simulink model "Unknown_Terrain_BOTS"  (R2018b)
settings: Solver=VariableStepAuto  StartTime=0.0  StopTime=10.0  RelTol=1e-3
model workspace: external: MATLAB File F:\Projects\Relative Localiztion\CAD models\Simulation\Unknown_Terrain_BOTS_DataFile.m (data not in the file)
values from neighbouring files (symbols this model uses):
  BOT1_pos = zeros(3,length(t))    [Tetrahedron_Based_Relative_Localization.m]
  bot1_transmitted = zeros(3,length(t))    [Transmission_Channal.m]
  BOT2_pos = zeros(3,length(t))    [Tetrahedron_Based_Relative_Localization.m]
  bot2_transmitted = zeros(3,length(t))    [Transmission_Channal.m]
  BOT3_pos = zeros(3,length(t))    [Tetrahedron_Based_Relative_Localization.m]
  bot3_transmitted = zeros(3,length(t))    [Transmission_Channal.m]
  BOT4_pos = zeros(3,length(t))    [Tetrahedron_Based_Relative_Localization.m]
  bot4_transmitted = zeros(3,length(t))    [Transmission_Channal.m]
undefined symbols (not defined in the file or in its folder): smiData, X, Y, Z
libraries: simulink x60, sm_lib x29, nesl_utility x25
(part 2 of 2)

== system Unknown_Terrain_BOTS/BOT1/BOT1_RIGID ==
  ReferenceFrame : sm_lib/Frames and Transforms/Reference Frame
  Solid : sm_lib/Body Elements/Solid  InertiaType=Custom  Mass=smiData.Solid(3).mass  MassUnits=kg  CenterOfMass=smiData.Solid(3).CoM  CenterOfMassUnits=mm  MomentsOfInertia=smiData.Solid(3).MoI  MomentsOfInertiaUnits=kg*mm^2  ProductsOfInertia=smiData.Solid(3).PoI  ProductsOfInertiaUnits=kg*mm^2  BasedOnType=Density  Density=1000  DensityUnits=kg/m^3  DoExposeReferenceFrame=on  SerializedFrames=<Frames/>  GraphicType=FromGeometry  MarkerShape=Sphere  MarkerSize=10  GraphicVisPropType=AdvancedVisualProperties  GraphicDiffuseColor=[1.0 0.2 0.2]  GraphicSpecularColor=[0.5 0.5 0.5 1.0]  GraphicAmbientColor=[0.15 0.15 0.15 1.0]  GraphicEmissiveColor=[0.0 0.0 0.0 1.0]  GraphicShininess=75  GraphicOpacity=smiData.Solid(3).opacity  GeometryShape=FromFile  RectangleSize=[1 1]  RectangleSizeUnits=m  BrickDimensions=[1 1 1]  BrickDimensionUnits=m  CylinderRadius=1  CylinderRadiusUnits=m  CylinderLength=1  CylinderLengthUnits=m  SphereRadius=1  SphereRadiusUnits=m  EllipsoidRadii=[1 1 1]  EllipsoidRadiiUnits=m  ExtrusionCrossSection=[1 1; -1 1; -1 -1; 1 -1]  ExtrusionCrossSectionUnits=m  ExtrusionLength=1  ExtrusionLengthUnits=m  PolygonNumSides=3  PolygonOuterRadius=1  PolygonOuterRadiusUnits=m  ExtGeomFileType=STEP  ExtGeomFileName=BOT3_Default_sldprt.STEP  ExtGeomFileUnits=m  RevolutionCrossSection=[1 1; 1 -1; 2 -1; 2 1]  RevolutionCrossSectionUnits=m  RevolutionExtent=Full  RevolutionAngle=180  RevolutionAngleUnits=deg
  Transform : sm_lib/Frames and Transforms/Rigid Transform  TranslationMethod=Cartesian  TranslationStandardOffset=0  TranslationLengthUnit=m  TranslationStandardAxis=+Z  TranslationCartesianOffset=smiData.RigidTransform(6).translation  TranslationROffset=0  TranslationROffsetUnits=m  TranslationZOffset=0  TranslationZOffsetUnits=m  TranslationThetaOffset=0  TranslationThetaOffsetUnits=deg  RotationMethod=ArbitraryAxis  RotationAngleUnits=rad  RotationStandardAxis=+Z  RotationAngle=smiData.RigidTransform(6).angle  RotationArbitraryAxis=smiData.RigidTransform(6).axis  FollAlignAxisA=+X  BaseAlignAxisA=+Y  FollAlignAxisB=+Y  BaseAlignAxisB=+Z  RotationSequenceAxes=FollowerAxes  RotationSequence=XYX  RotationSequenceAngles=[0 0 0]  RotationSequenceAnglesUnits=deg  RotationMatrix=[1 0 0; 0 1 0; 0 0 1]
  F : PMIOPort  Side=Left
  connections:
  Solid/RConn1 -- ReferenceFrame/RConn1 -- Transform/LConn1
  Transform/RConn1 -- F/RConn1

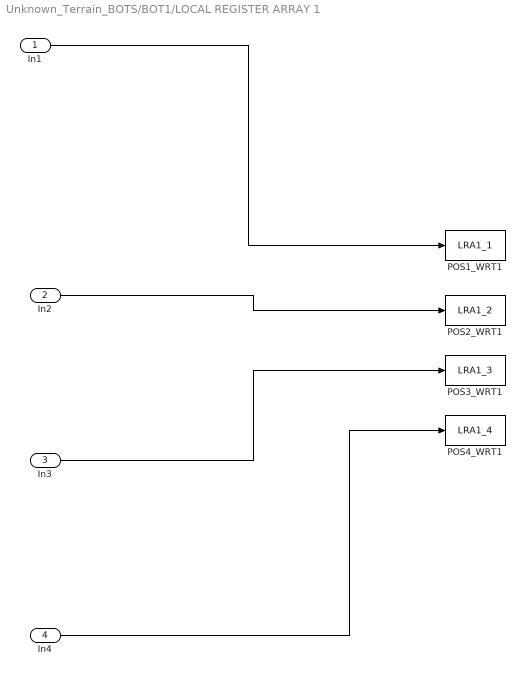
== system Unknown_Terrain_BOTS/BOT1/LOCAL REGISTER ARRAY 1 ==
  In1 : Inport
  In2 : Inport  Port=2
  In3 : Inport  Port=3
  In4 : Inport  Port=4
  POS1_WRT1 : ToWorkspace  VariableName=LRA1_1  SampleTime=-1
  POS2_WRT1 : ToWorkspace  VariableName=LRA1_2  SampleTime=-1
  POS3_WRT1 : ToWorkspace  VariableName=LRA1_3  SampleTime=-1
  POS4_WRT1 : ToWorkspace  VariableName=LRA1_4  SampleTime=-1
  wires:
  In2/1 -> POS2_WRT1/1
  In3/1 -> POS3_WRT1/1
  In1/1 -> POS1_WRT1/1
  In4/1 -> POS4_WRT1/1

== system Unknown_Terrain_BOTS/BOT1/Subsystem ==
  1 : Inport
  Gain : Gain  Gain=-1
  Sum : Sum  Inputs=|++
  z0 : Constant  Value=0.2889717
  2 : Outport
  wires:
  z0/1 -> Sum/2
  Gain/1 -> Sum/1
  Sum/1 -> 2/1
  1/1 -> Gain/1

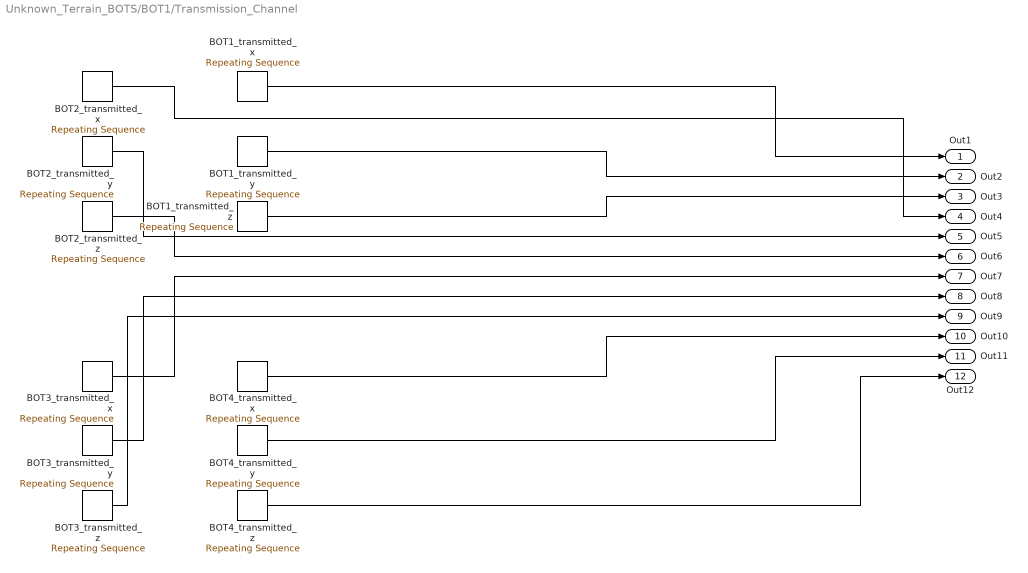
== system Unknown_Terrain_BOTS/BOT1/Transmission_Channel ==
  BOT1_transmitted_x : simulink/Sources/Repeating Sequence  rep_seq_t=t  rep_seq_y=bot1_transmitted(1,:)
  BOT1_transmitted_y : simulink/Sources/Repeating Sequence  rep_seq_t=t  rep_seq_y=bot1_transmitted(2,:)
  BOT1_transmitted_z : simulink/Sources/Repeating Sequence  rep_seq_t=t  rep_seq_y=bot1_transmitted(3,:)
  BOT2_transmitted_x : simulink/Sources/Repeating Sequence  rep_seq_t=t  rep_seq_y=bot2_transmitted(1,:)
  BOT2_transmitted_y : simulink/Sources/Repeating Sequence  rep_seq_t=t  rep_seq_y=bot2_transmitted(2,:)
  BOT2_transmitted_z : simulink/Sources/Repeating Sequence  rep_seq_t=t  rep_seq_y=bot2_transmitted(3,:)
  BOT3_transmitted_x : simulink/Sources/Repeating Sequence  rep_seq_t=t  rep_seq_y=bot3_transmitted(1,:)
  BOT3_transmitted_y : simulink/Sources/Repeating Sequence  rep_seq_t=t  rep_seq_y=bot3_transmitted(2,:)
  BOT3_transmitted_z : simulink/Sources/Repeating Sequence  rep_seq_t=t  rep_seq_y=bot3_transmitted(3,:)
  BOT4_transmitted_x : simulink/Sources/Repeating Sequence  rep_seq_t=t  rep_seq_y=bot4_transmitted(1,:)
  BOT4_transmitted_y : simulink/Sources/Repeating Sequence  rep_seq_t=t  rep_seq_y=bot4_transmitted(2,:)
  BOT4_transmitted_z : simulink/Sources/Repeating Sequence  rep_seq_t=t  rep_seq_y=bot4_transmitted(3,:)
  Out1 : Outport
  Out2 : Outport  Port=2
  Out3 : Outport  Port=3
  Out4 : Outport  Port=4
  Out5 : Outport  Port=5
  Out6 : Outport  Port=6
  Out7 : Outport  Port=7
  Out8 : Outport  Port=8
  Out9 : Outport  Port=9
  Out10 : Outport  Port=10
  Out11 : Outport  Port=11
  Out12 : Outport  Port=12
  wires:
  BOT1_transmitted_x/1 -> Out1/1
  BOT4_transmitted_z/1 -> Out12/1
  BOT1_transmitted_z/1 -> Out3/1
  BOT3_transmitted_x/1 -> Out7/1
  BOT3_transmitted_z/1 -> Out9/1
  BOT2_transmitted_z/1 -> Out6/1
  BOT2_transmitted_y/1 -> Out5/1
  BOT3_transmitted_y/1 -> Out8/1
  BOT1_transmitted_y/1 -> Out2/1
  BOT2_transmitted_x/1 -> Out4/1
  BOT4_transmitted_x/1 -> Out10/1
  BOT4_transmitted_y/1 -> Out11/1

== system Unknown_Terrain_BOTS/BOT2/BOT2_RIGID ==
  ReferenceFrame : sm_lib/Frames and Transforms/Reference Frame
  Solid : sm_lib/Body Elements/Solid  InertiaType=Custom  Mass=smiData.Solid(4).mass  MassUnits=kg  CenterOfMass=smiData.Solid(4).CoM  CenterOfMassUnits=mm  MomentsOfInertia=smiData.Solid(4).MoI  MomentsOfInertiaUnits=kg*mm^2  ProductsOfInertia=smiData.Solid(4).PoI  ProductsOfInertiaUnits=kg*mm^2  BasedOnType=Density  Density=1000  DensityUnits=kg/m^3  DoExposeReferenceFrame=on  SerializedFrames=<Frames/>  GraphicType=FromGeometry  MarkerShape=Sphere  MarkerSize=10  GraphicVisPropType=AdvancedVisualProperties  GraphicDiffuseColor=[0.6 1.0 0.2]  GraphicSpecularColor=[0.5 0.5 0.5 1.0]  GraphicAmbientColor=[0.15 0.15 0.15 1.0]  GraphicEmissiveColor=[0.0 0.0 0.0 1.0]  GraphicShininess=75  GraphicOpacity=smiData.Solid(4).opacity  GeometryShape=FromFile  RectangleSize=[1 1]  RectangleSizeUnits=m  BrickDimensions=[1 1 1]  BrickDimensionUnits=m  CylinderRadius=1  CylinderRadiusUnits=m  CylinderLength=1  CylinderLengthUnits=m  SphereRadius=1  SphereRadiusUnits=m  EllipsoidRadii=[1 1 1]  EllipsoidRadiiUnits=m  ExtrusionCrossSection=[1 1; -1 1; -1 -1; 1 -1]  ExtrusionCrossSectionUnits=m  ExtrusionLength=1  ExtrusionLengthUnits=m  PolygonNumSides=3  PolygonOuterRadius=1  PolygonOuterRadiusUnits=m  ExtGeomFileType=STEP  ExtGeomFileName=BOT4_Default_sldprt.STEP  ExtGeomFileUnits=m  RevolutionCrossSection=[1 1; 1 -1; 2 -1; 2 1]  RevolutionCrossSectionUnits=m  RevolutionExtent=Full  RevolutionAngle=180  RevolutionAngleUnits=deg
  Transform : sm_lib/Frames and Transforms/Rigid Transform  TranslationMethod=Cartesian  TranslationStandardOffset=0  TranslationLengthUnit=m  TranslationStandardAxis=+Z  TranslationCartesianOffset=smiData.RigidTransform(8).translation  TranslationROffset=0  TranslationROffsetUnits=m  TranslationZOffset=0  TranslationZOffsetUnits=m  TranslationThetaOffset=0  TranslationThetaOffsetUnits=deg  RotationMethod=ArbitraryAxis  RotationAngleUnits=rad  RotationStandardAxis=+Z  RotationAngle=smiData.RigidTransform(8).angle  RotationArbitraryAxis=smiData.RigidTransform(8).axis  FollAlignAxisA=+X  BaseAlignAxisA=+Y  FollAlignAxisB=+Y  BaseAlignAxisB=+Z  RotationSequenceAxes=FollowerAxes  RotationSequence=XYX  RotationSequenceAngles=[0 0 0]  RotationSequenceAnglesUnits=deg  RotationMatrix=[1 0 0; 0 1 0; 0 0 1]
  F : PMIOPort  Side=Left
  connections:
  Solid/RConn1 -- ReferenceFrame/RConn1 -- Transform/LConn1
  Transform/RConn1 -- F/RConn1

== system Unknown_Terrain_BOTS/BOT2/LOCAL REGISTER ARRAY 2 ==
  In1 : Inport
  In2 : Inport  Port=2
  In3 : Inport  Port=3
  In4 : Inport  Port=4
  POS1_WRT2 : ToWorkspace  VariableName=LRA2_1  SampleTime=-1
  POS2_WRT2 : ToWorkspace  VariableName=LRA2_2  SampleTime=-1
  POS3_WRT2 : ToWorkspace  VariableName=LRA2_3  SampleTime=-1
  POS4_WRT2 : ToWorkspace  VariableName=LRA2_4  SampleTime=-1
  wires:
  In2/1 -> POS2_WRT2/1
  In3/1 -> POS3_WRT2/1
  In1/1 -> POS1_WRT2/1
  In4/1 -> POS4_WRT2/1

== system Unknown_Terrain_BOTS/BOT2/Subsystem ==
  1 : Inport
  Gain : Gain
  Sum : Sum  Inputs=|++
  z0 : Constant  Value=-0.2889717
  2 : Outport
  wires:
  z0/1 -> Sum/2
  Gain/1 -> Sum/1
  Sum/1 -> 2/1
  1/1 -> Gain/1

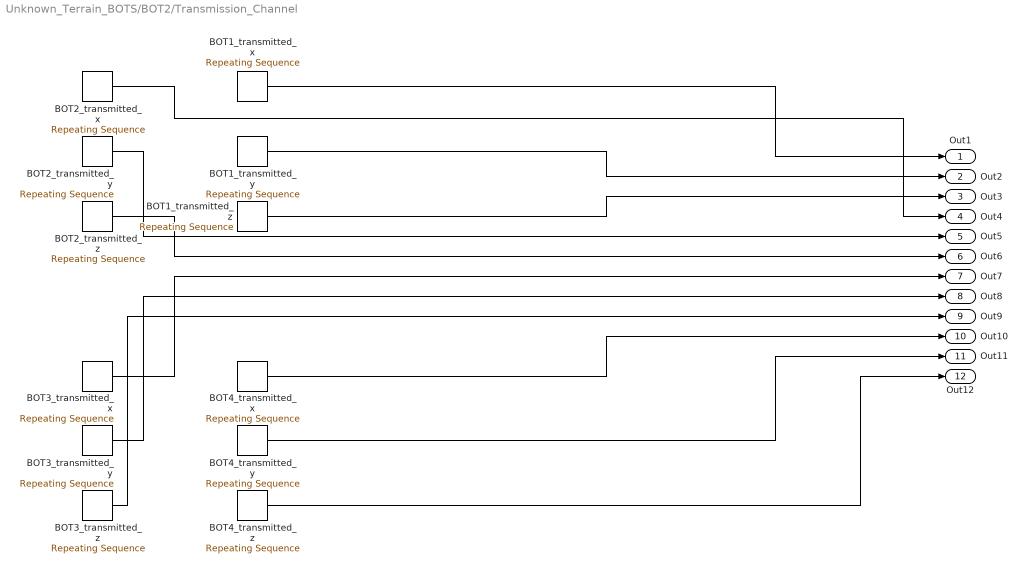
== system Unknown_Terrain_BOTS/BOT2/Transmission_Channel ==
  BOT1_transmitted_x : simulink/Sources/Repeating Sequence  rep_seq_t=t  rep_seq_y=bot1_transmitted(1,:)
  BOT1_transmitted_y : simulink/Sources/Repeating Sequence  rep_seq_t=t  rep_seq_y=bot1_transmitted(2,:)
  BOT1_transmitted_z : simulink/Sources/Repeating Sequence  rep_seq_t=t  rep_seq_y=bot1_transmitted(3,:)
  BOT2_transmitted_x : simulink/Sources/Repeating Sequence  rep_seq_t=t  rep_seq_y=bot2_transmitted(1,:)
  BOT2_transmitted_y : simulink/Sources/Repeating Sequence  rep_seq_t=t  rep_seq_y=bot2_transmitted(2,:)
  BOT2_transmitted_z : simulink/Sources/Repeating Sequence  rep_seq_t=t  rep_seq_y=bot2_transmitted(3,:)
  BOT3_transmitted_x : simulink/Sources/Repeating Sequence  rep_seq_t=t  rep_seq_y=bot3_transmitted(1,:)
  BOT3_transmitted_y : simulink/Sources/Repeating Sequence  rep_seq_t=t  rep_seq_y=bot3_transmitted(2,:)
  BOT3_transmitted_z : simulink/Sources/Repeating Sequence  rep_seq_t=t  rep_seq_y=bot3_transmitted(3,:)
  BOT4_transmitted_x : simulink/Sources/Repeating Sequence  rep_seq_t=t  rep_seq_y=bot4_transmitted(1,:)
  BOT4_transmitted_y : simulink/Sources/Repeating Sequence  rep_seq_t=t  rep_seq_y=bot4_transmitted(2,:)
  BOT4_transmitted_z : simulink/Sources/Repeating Sequence  rep_seq_t=t  rep_seq_y=bot4_transmitted(3,:)
  Out1 : Outport
  Out2 : Outport  Port=2
  Out3 : Outport  Port=3
  Out4 : Outport  Port=4
  Out5 : Outport  Port=5
  Out6 : Outport  Port=6
  Out7 : Outport  Port=7
  Out8 : Outport  Port=8
  Out9 : Outport  Port=9
  Out10 : Outport  Port=10
  Out11 : Outport  Port=11
  Out12 : Outport  Port=12
  wires:
  BOT1_transmitted_x/1 -> Out1/1
  BOT4_transmitted_z/1 -> Out12/1
  BOT1_transmitted_z/1 -> Out3/1
  BOT3_transmitted_x/1 -> Out7/1
  BOT3_transmitted_z/1 -> Out9/1
  BOT2_transmitted_z/1 -> Out6/1
  BOT2_transmitted_y/1 -> Out5/1
  BOT3_transmitted_y/1 -> Out8/1
  BOT1_transmitted_y/1 -> Out2/1
  BOT2_transmitted_x/1 -> Out4/1
  BOT4_transmitted_x/1 -> Out10/1
  BOT4_transmitted_y/1 -> Out11/1

== system Unknown_Terrain_BOTS/BOT3/BOT3_RIGID ==
  ReferenceFrame : sm_lib/Frames and Transforms/Reference Frame
  Solid : sm_lib/Body Elements/Solid  InertiaType=Custom  Mass=smiData.Solid(2).mass  MassUnits=kg  CenterOfMass=smiData.Solid(2).CoM  CenterOfMassUnits=mm  MomentsOfInertia=smiData.Solid(2).MoI  MomentsOfInertiaUnits=kg*mm^2  ProductsOfInertia=smiData.Solid(2).PoI  ProductsOfInertiaUnits=kg*mm^2  BasedOnType=Density  Density=1000  DensityUnits=kg/m^3  DoExposeReferenceFrame=on  SerializedFrames=<Frames/>  GraphicType=FromGeometry  MarkerShape=Sphere  MarkerSize=10  GraphicVisPropType=AdvancedVisualProperties  GraphicDiffuseColor=[0.0 0.2 1.0]  GraphicSpecularColor=[0.5 0.5 0.5 1.0]  GraphicAmbientColor=[0.15 0.15 0.15 1.0]  GraphicEmissiveColor=[0.0 0.0 0.0 1.0]  GraphicShininess=75  GraphicOpacity=smiData.Solid(2).opacity  GeometryShape=FromFile  RectangleSize=[1 1]  RectangleSizeUnits=m  BrickDimensions=[1 1 1]  BrickDimensionUnits=m  CylinderRadius=1  CylinderRadiusUnits=m  CylinderLength=1  CylinderLengthUnits=m  SphereRadius=1  SphereRadiusUnits=m  EllipsoidRadii=[1 1 1]  EllipsoidRadiiUnits=m  ExtrusionCrossSection=[1 1; -1 1; -1 -1; 1 -1]  ExtrusionCrossSectionUnits=m  ExtrusionLength=1  ExtrusionLengthUnits=m  PolygonNumSides=3  PolygonOuterRadius=1  PolygonOuterRadiusUnits=m  ExtGeomFileType=STEP  ExtGeomFileName=BOT2_Default_sldprt.STEP  ExtGeomFileUnits=m  RevolutionCrossSection=[1 1; 1 -1; 2 -1; 2 1]  RevolutionCrossSectionUnits=m  RevolutionExtent=Full  RevolutionAngle=180  RevolutionAngleUnits=deg
  Transform : sm_lib/Frames and Transforms/Rigid Transform  TranslationMethod=Cartesian  TranslationStandardOffset=0  TranslationLengthUnit=m  TranslationStandardAxis=+Z  TranslationCartesianOffset=smiData.RigidTransform(4).translation  TranslationROffset=0  TranslationROffsetUnits=m  TranslationZOffset=0  TranslationZOffsetUnits=m  TranslationThetaOffset=0  TranslationThetaOffsetUnits=deg  RotationMethod=ArbitraryAxis  RotationAngleUnits=rad  RotationStandardAxis=+Z  RotationAngle=smiData.RigidTransform(4).angle  RotationArbitraryAxis=smiData.RigidTransform(4).axis  FollAlignAxisA=+X  BaseAlignAxisA=+Y  FollAlignAxisB=+Y  BaseAlignAxisB=+Z  RotationSequenceAxes=FollowerAxes  RotationSequence=XYX  RotationSequenceAngles=[0 0 0]  RotationSequenceAnglesUnits=deg  RotationMatrix=[1 0 0; 0 1 0; 0 0 1]
  F : PMIOPort  Side=Left
  connections:
  Solid/RConn1 -- ReferenceFrame/RConn1 -- Transform/LConn1
  Transform/RConn1 -- F/RConn1

== system Unknown_Terrain_BOTS/BOT3/LOCAL REGISTER ARRAY 3 ==
  In1 : Inport
  In2 : Inport  Port=2
  In3 : Inport  Port=3
  In4 : Inport  Port=4
  POS1_WRT3 : ToWorkspace  VariableName=LRA3_1  SampleTime=-1
  POS2_WRT3 : ToWorkspace  VariableName=LRA3_2  SampleTime=-1
  POS3_WRT3 : ToWorkspace  VariableName=LRA3_3  SampleTime=-1
  POS4_WRT3 : ToWorkspace  VariableName=LRA3_4  SampleTime=-1
  wires:
  In2/1 -> POS2_WRT3/1
  In3/1 -> POS3_WRT3/1
  In1/1 -> POS1_WRT3/1
  In4/1 -> POS4_WRT3/1

== system Unknown_Terrain_BOTS/BOT3/Subsystem ==
  1 : Inport
  Gain : Gain
  Sum : Sum  Inputs=|++
  z0 : Constant  Value=-0.2889717
  2 : Outport
  wires:
  z0/1 -> Sum/2
  Gain/1 -> Sum/1
  Sum/1 -> 2/1
  1/1 -> Gain/1

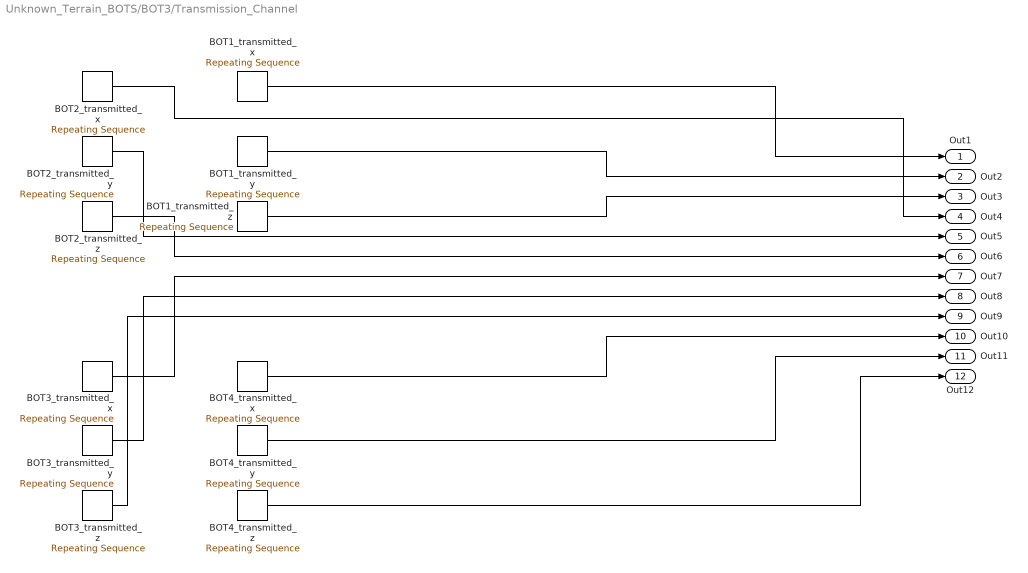
== system Unknown_Terrain_BOTS/BOT3/Transmission_Channel ==
  BOT1_transmitted_x : simulink/Sources/Repeating Sequence  rep_seq_t=t  rep_seq_y=bot1_transmitted(1,:)
  BOT1_transmitted_y : simulink/Sources/Repeating Sequence  rep_seq_t=t  rep_seq_y=bot1_transmitted(2,:)
  BOT1_transmitted_z : simulink/Sources/Repeating Sequence  rep_seq_t=t  rep_seq_y=bot1_transmitted(3,:)
  BOT2_transmitted_x : simulink/Sources/Repeating Sequence  rep_seq_t=t  rep_seq_y=bot2_transmitted(1,:)
  BOT2_transmitted_y : simulink/Sources/Repeating Sequence  rep_seq_t=t  rep_seq_y=bot2_transmitted(2,:)
  BOT2_transmitted_z : simulink/Sources/Repeating Sequence  rep_seq_t=t  rep_seq_y=bot2_transmitted(3,:)
  BOT3_transmitted_x : simulink/Sources/Repeating Sequence  rep_seq_t=t  rep_seq_y=bot3_transmitted(1,:)
  BOT3_transmitted_y : simulink/Sources/Repeating Sequence  rep_seq_t=t  rep_seq_y=bot3_transmitted(2,:)
  BOT3_transmitted_z : simulink/Sources/Repeating Sequence  rep_seq_t=t  rep_seq_y=bot3_transmitted(3,:)
  BOT4_transmitted_x : simulink/Sources/Repeating Sequence  rep_seq_t=t  rep_seq_y=bot4_transmitted(1,:)
  BOT4_transmitted_y : simulink/Sources/Repeating Sequence  rep_seq_t=t  rep_seq_y=bot4_transmitted(2,:)
  BOT4_transmitted_z : simulink/Sources/Repeating Sequence  rep_seq_t=t  rep_seq_y=bot4_transmitted(3,:)
  Out1 : Outport
  Out2 : Outport  Port=2
  Out3 : Outport  Port=3
  Out4 : Outport  Port=4
  Out5 : Outport  Port=5
  Out6 : Outport  Port=6
  Out7 : Outport  Port=7
  Out8 : Outport  Port=8
  Out9 : Outport  Port=9
  Out10 : Outport  Port=10
  Out11 : Outport  Port=11
  Out12 : Outport  Port=12
  wires:
  BOT1_transmitted_x/1 -> Out1/1
  BOT4_transmitted_z/1 -> Out12/1
  BOT1_transmitted_z/1 -> Out3/1
  BOT3_transmitted_x/1 -> Out7/1
  BOT3_transmitted_z/1 -> Out9/1
  BOT2_transmitted_z/1 -> Out6/1
  BOT2_transmitted_y/1 -> Out5/1
  BOT3_transmitted_y/1 -> Out8/1
  BOT1_transmitted_y/1 -> Out2/1
  BOT2_transmitted_x/1 -> Out4/1
  BOT4_transmitted_x/1 -> Out10/1
  BOT4_transmitted_y/1 -> Out11/1

== system Unknown_Terrain_BOTS/BOT4/BOT4_RIGID ==
  ReferenceFrame : sm_lib/Frames and Transforms/Reference Frame
  Solid : sm_lib/Body Elements/Solid  InertiaType=Custom  Mass=smiData.Solid(1).mass  MassUnits=kg  CenterOfMass=smiData.Solid(1).CoM  CenterOfMassUnits=mm  MomentsOfInertia=smiData.Solid(1).MoI  MomentsOfInertiaUnits=kg*mm^2  ProductsOfInertia=smiData.Solid(1).PoI  ProductsOfInertiaUnits=kg*mm^2  BasedOnType=Density  Density=1000  DensityUnits=kg/m^3  DoExposeReferenceFrame=on  SerializedFrames=<Frames/>  GraphicType=FromGeometry  MarkerShape=Sphere  MarkerSize=10  GraphicVisPropType=AdvancedVisualProperties  GraphicDiffuseColor=[0.4 0.4 0.4]  GraphicSpecularColor=[0.5 0.5 0.5 1.0]  GraphicAmbientColor=[0.15 0.15 0.15 1.0]  GraphicEmissiveColor=[0.0 0.0 0.0 1.0]  GraphicShininess=75  GraphicOpacity=smiData.Solid(1).opacity  GeometryShape=FromFile  RectangleSize=[1 1]  RectangleSizeUnits=m  BrickDimensions=[1 1 1]  BrickDimensionUnits=m  CylinderRadius=1  CylinderRadiusUnits=m  CylinderLength=1  CylinderLengthUnits=m  SphereRadius=1  SphereRadiusUnits=m  EllipsoidRadii=[1 1 1]  EllipsoidRadiiUnits=m  ExtrusionCrossSection=[1 1; -1 1; -1 -1; 1 -1]  ExtrusionCrossSectionUnits=m  ExtrusionLength=1  ExtrusionLengthUnits=m  PolygonNumSides=3  PolygonOuterRadius=1  PolygonOuterRadiusUnits=m  ExtGeomFileType=STEP  ExtGeomFileName=BOT1_Default_sldprt.STEP  ExtGeomFileUnits=m  RevolutionCrossSection=[1 1; 1 -1; 2 -1; 2 1]  RevolutionCrossSectionUnits=m  RevolutionExtent=Full  RevolutionAngle=180  RevolutionAngleUnits=deg
  Transform : sm_lib/Frames and Transforms/Rigid Transform  TranslationMethod=Cartesian  TranslationStandardOffset=0  TranslationLengthUnit=m  TranslationStandardAxis=+Z  TranslationCartesianOffset=smiData.RigidTransform(2).translation  TranslationROffset=0  TranslationROffsetUnits=m  TranslationZOffset=0  TranslationZOffsetUnits=m  TranslationThetaOffset=0  TranslationThetaOffsetUnits=deg  RotationMethod=ArbitraryAxis  RotationAngleUnits=rad  RotationStandardAxis=+Z  RotationAngle=smiData.RigidTransform(2).angle  RotationArbitraryAxis=smiData.RigidTransform(2).axis  FollAlignAxisA=+X  BaseAlignAxisA=+Y  FollAlignAxisB=+Y  BaseAlignAxisB=+Z  RotationSequenceAxes=FollowerAxes  RotationSequence=XYX  RotationSequenceAngles=[0 0 0]  RotationSequenceAnglesUnits=deg  RotationMatrix=[1 0 0; 0 1 0; 0 0 1]
  F : PMIOPort  Side=Left
  connections:
  Solid/RConn1 -- ReferenceFrame/RConn1 -- Transform/LConn1
  Transform/RConn1 -- F/RConn1

== system Unknown_Terrain_BOTS/BOT4/LOCAL REGISTER ARRAY 4 ==
  In1 : Inport
  In2 : Inport  Port=2
  In3 : Inport  Port=3
  In4 : Inport  Port=4
  POS1_WRT4 : ToWorkspace  VariableName=LRA4_1  SampleTime=-1
  POS2_WRT4 : ToWorkspace  VariableName=LRA4_2  SampleTime=-1
  POS3_WRT4 : ToWorkspace  VariableName=LRA4_3  SampleTime=-1
  POS4_WRT4 : ToWorkspace  VariableName=LRA4_4  SampleTime=-1
  wires:
  In2/1 -> POS2_WRT4/1
  In3/1 -> POS3_WRT4/1
  In1/1 -> POS1_WRT4/1
  In4/1 -> POS4_WRT4/1

== system Unknown_Terrain_BOTS/BOT4/Subsystem ==
  1 : Inport
  Gain : Gain
  Sum : Sum  Inputs=|++
  z0 : Constant  Value=-0.2889717
  2 : Outport
  wires:
  z0/1 -> Sum/2
  Gain/1 -> Sum/1
  Sum/1 -> 2/1
  1/1 -> Gain/1

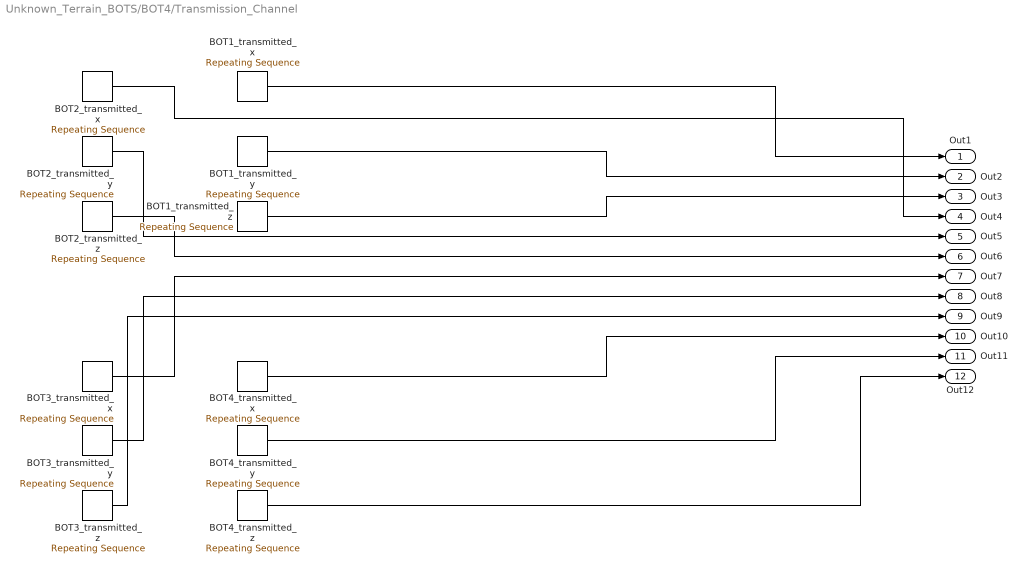
== system Unknown_Terrain_BOTS/BOT4/Transmission_Channel ==
  BOT1_transmitted_x : simulink/Sources/Repeating Sequence  rep_seq_t=t  rep_seq_y=bot1_transmitted(1,:)
  BOT1_transmitted_y : simulink/Sources/Repeating Sequence  rep_seq_t=t  rep_seq_y=bot1_transmitted(2,:)
  BOT1_transmitted_z : simulink/Sources/Repeating Sequence  rep_seq_t=t  rep_seq_y=bot1_transmitted(3,:)
  BOT2_transmitted_x : simulink/Sources/Repeating Sequence  rep_seq_t=t  rep_seq_y=bot2_transmitted(1,:)
  BOT2_transmitted_y : simulink/Sources/Repeating Sequence  rep_seq_t=t  rep_seq_y=bot2_transmitted(2,:)
  BOT2_transmitted_z : simulink/Sources/Repeating Sequence  rep_seq_t=t  rep_seq_y=bot2_transmitted(3,:)
  BOT3_transmitted_x : simulink/Sources/Repeating Sequence  rep_seq_t=t  rep_seq_y=bot3_transmitted(1,:)
  BOT3_transmitted_y : simulink/Sources/Repeating Sequence  rep_seq_t=t  rep_seq_y=bot3_transmitted(2,:)
  BOT3_transmitted_z : simulink/Sources/Repeating Sequence  rep_seq_t=t  rep_seq_y=bot3_transmitted(3,:)
  BOT4_transmitted_x : simulink/Sources/Repeating Sequence  rep_seq_t=t  rep_seq_y=bot4_transmitted(1,:)
  BOT4_transmitted_y : simulink/Sources/Repeating Sequence  rep_seq_t=t  rep_seq_y=bot4_transmitted(2,:)
  BOT4_transmitted_z : simulink/Sources/Repeating Sequence  rep_seq_t=t  rep_seq_y=bot4_transmitted(3,:)
  Out1 : Outport
  Out2 : Outport  Port=2
  Out3 : Outport  Port=3
  Out4 : Outport  Port=4
  Out5 : Outport  Port=5
  Out6 : Outport  Port=6
  Out7 : Outport  Port=7
  Out8 : Outport  Port=8
  Out9 : Outport  Port=9
  Out10 : Outport  Port=10
  Out11 : Outport  Port=11
  Out12 : Outport  Port=12
  wires:
  BOT1_transmitted_x/1 -> Out1/1
  BOT4_transmitted_z/1 -> Out12/1
  BOT1_transmitted_z/1 -> Out3/1
  BOT3_transmitted_x/1 -> Out7/1
  BOT3_transmitted_z/1 -> Out9/1
  BOT2_transmitted_z/1 -> Out6/1
  BOT2_transmitted_y/1 -> Out5/1
  BOT3_transmitted_y/1 -> Out8/1
  BOT1_transmitted_y/1 -> Out2/1
  BOT2_transmitted_x/1 -> Out4/1
  BOT4_transmitted_x/1 -> Out10/1
  BOT4_transmitted_y/1 -> Out11/1

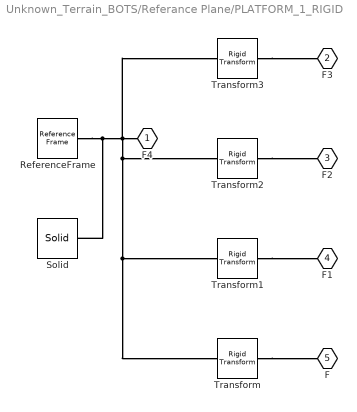
== system Unknown_Terrain_BOTS/Referance Plane/PLATFORM_1_RIGID ==
  ReferenceFrame : sm_lib/Frames and Transforms/Reference Frame
  Solid : sm_lib/Body Elements/Solid  InertiaType=Custom  Mass=smiData.Solid(5).mass  MassUnits=kg  CenterOfMass=smiData.Solid(5).CoM  CenterOfMassUnits=mm  MomentsOfInertia=smiData.Solid(5).MoI  MomentsOfInertiaUnits=kg*mm^2  ProductsOfInertia=smiData.Solid(5).PoI  ProductsOfInertiaUnits=kg*mm^2  BasedOnType=Density  Density=1000  DensityUnits=kg/m^3  DoExposeReferenceFrame=on  SerializedFrames=<Frames/>  GraphicType=FromGeometry  MarkerShape=Sphere  MarkerSize=10  GraphicVisPropType=SimpleVisualProperties  GraphicDiffuseColor=smiData.Solid(5).color  GraphicSpecularColor=[0.5 0.5 0.5 1.0]  GraphicAmbientColor=[0.15 0.15 0.15 1.0]  GraphicEmissiveColor=[0.0 0.0 0.0 1.0]  GraphicShininess=75  GraphicOpacity=smiData.Solid(5).opacity  GeometryShape=FromFile  RectangleSize=[1 1]  RectangleSizeUnits=m  BrickDimensions=[1 1 1]  BrickDimensionUnits=m  CylinderRadius=1  CylinderRadiusUnits=m  CylinderLength=1  CylinderLengthUnits=m  SphereRadius=1  SphereRadiusUnits=m  EllipsoidRadii=[1 1 1]  EllipsoidRadiiUnits=m  ExtrusionCrossSection=[1 1; -1 1; -1 -1; 1 -1]  ExtrusionCrossSectionUnits=m  ExtrusionLength=1  ExtrusionLengthUnits=m  PolygonNumSides=3  PolygonOuterRadius=1  PolygonOuterRadiusUnits=m  ExtGeomFileType=STEP  ExtGeomFileName=PLATFORM_Default_sldprt.STEP  ExtGeomFileUnits=m  RevolutionCrossSection=[1 1; 1 -1; 2 -1; 2 1]  RevolutionCrossSectionUnits=m  RevolutionExtent=Full  RevolutionAngle=180  RevolutionAngleUnits=deg
  Transform : sm_lib/Frames and Transforms/Rigid Transform  TranslationMethod=Cartesian  TranslationStandardOffset=0  TranslationLengthUnit=m  TranslationStandardAxis=+Z  TranslationCartesianOffset=smiData.RigidTransform(1).translation  TranslationROffset=0  TranslationROffsetUnits=m  TranslationZOffset=0  TranslationZOffsetUnits=m  TranslationThetaOffset=0  TranslationThetaOffsetUnits=deg  RotationMethod=ArbitraryAxis  RotationAngleUnits=rad  RotationStandardAxis=+Z  RotationAngle=smiData.RigidTransform(1).angle  RotationArbitraryAxis=smiData.RigidTransform(1).axis  FollAlignAxisA=+X  BaseAlignAxisA=+Y  FollAlignAxisB=+Y  BaseAlignAxisB=+Z  RotationSequenceAxes=FollowerAxes  RotationSequence=XYX  RotationSequenceAngles=[0 0 0]  RotationSequenceAnglesUnits=deg  RotationMatrix=[1 0 0; 0 1 0; 0 0 1]
  Transform1 : sm_lib/Frames and Transforms/Rigid Transform  TranslationMethod=Cartesian  TranslationStandardOffset=0  TranslationLengthUnit=m  TranslationStandardAxis=+Z  TranslationCartesianOffset=smiData.RigidTransform(3).translation  TranslationROffset=0  TranslationROffsetUnits=m  TranslationZOffset=0  TranslationZOffsetUnits=m  TranslationThetaOffset=0  TranslationThetaOffsetUnits=deg  RotationMethod=ArbitraryAxis  RotationAngleUnits=rad  RotationStandardAxis=+Z  RotationAngle=smiData.RigidTransform(3).angle  RotationArbitraryAxis=smiData.RigidTransform(3).axis  FollAlignAxisA=+X  BaseAlignAxisA=+Y  FollAlignAxisB=+Y  BaseAlignAxisB=+Z  RotationSequenceAxes=FollowerAxes  RotationSequence=XYX  RotationSequenceAngles=[0 0 0]  RotationSequenceAnglesUnits=deg  RotationMatrix=[1 0 0; 0 1 0; 0 0 1]
  Transform2 : sm_lib/Frames and Transforms/Rigid Transform  TranslationMethod=Cartesian  TranslationStandardOffset=0  TranslationLengthUnit=m  TranslationStandardAxis=+Z  TranslationCartesianOffset=smiData.RigidTransform(5).translation  TranslationROffset=0  TranslationROffsetUnits=m  TranslationZOffset=0  TranslationZOffsetUnits=m  TranslationThetaOffset=0  TranslationThetaOffsetUnits=deg  RotationMethod=ArbitraryAxis  RotationAngleUnits=rad  RotationStandardAxis=+Z  RotationAngle=smiData.RigidTransform(5).angle  RotationArbitraryAxis=smiData.RigidTransform(5).axis  FollAlignAxisA=+X  BaseAlignAxisA=+Y  FollAlignAxisB=+Y  BaseAlignAxisB=+Z  RotationSequenceAxes=FollowerAxes  RotationSequence=XYX  RotationSequenceAngles=[0 0 0]  RotationSequenceAnglesUnits=deg  RotationMatrix=[1 0 0; 0 1 0; 0 0 1]
  Transform3 : sm_lib/Frames and Transforms/Rigid Transform  TranslationMethod=Cartesian  TranslationStandardOffset=0  TranslationLengthUnit=m  TranslationStandardAxis=+Z  TranslationCartesianOffset=smiData.RigidTransform(7).translation  TranslationROffset=0  TranslationROffsetUnits=m  TranslationZOffset=0  TranslationZOffsetUnits=m  TranslationThetaOffset=0  TranslationThetaOffsetUnits=deg  RotationMethod=ArbitraryAxis  RotationAngleUnits=rad  RotationStandardAxis=+Z  RotationAngle=smiData.RigidTransform(7).angle  RotationArbitraryAxis=smiData.RigidTransform(7).axis  FollAlignAxisA=+X  BaseAlignAxisA=+Y  FollAlignAxisB=+Y  BaseAlignAxisB=+Z  RotationSequenceAxes=FollowerAxes  RotationSequence=XYX  RotationSequenceAngles=[0 0 0]  RotationSequenceAnglesUnits=deg  RotationMatrix=[1 0 0; 0 1 0; 0 0 1]
  F4 : PMIOPort  Side=Left
  F3 : PMIOPort  Port=2  Side=Right
  F2 : PMIOPort  Port=3  Side=Right
  F1 : PMIOPort  Port=4  Side=Right
  F : PMIOPort  Port=5  Side=Right
  connections:
  Solid/RConn1 -- ReferenceFrame/RConn1 -- Transform/LConn1 -- Transform1/LConn1 -- Transform2/LConn1 -- Transform3/LConn1 -- F4/RConn1
  Transform/RConn1 -- F/RConn1
  Transform1/RConn1 -- F1/RConn1
  Transform2/RConn1 -- F2/RConn1
  Transform3/RConn1 -- F3/RConn1

== matlab function Unknown_Terrain_BOTS/BOT4/Pose Estimator Bot1 ==
  data: x output; r1t input; y output; r2t input; r3t input; r4t input; z output
function [x,y,z] = fcn(r1t,r2t,r3t,r4t)
M = [0 -3.8462 0;4.4412 2.2206 0;-1.5702 -3.3140 -4.7104];
R = [r2t^2-r1t^2;r3t^2-r2t^2;r4t^2-r3t^2];
P = M*R;
x = P(1);
y = P(2);
z = P(3);

== matlab function Unknown_Terrain_BOTS/BOT4/Pose Estimator Bot2 ==
  data: x output; r1t input; y output; r2t input; r3t input; r4t input; z output
function [x,y,z] = fcn(r1t,r2t,r3t,r4t)
M = [0 -3.8462 0;4.4412 2.2206 0;-1.5702 -3.3140 -4.7104];
R = [r2t^2-r1t^2;r3t^2-r2t^2;r4t^2-r3t^2];
P = M*R;
x = P(1);
y = P(2);
z = P(3);

== matlab function Unknown_Terrain_BOTS/BOT4/Pose Estimator Bot3 ==
  data: x output; r1t input; y output; r2t input; r3t input; r4t input; z output
function [x,y,z] = fcn(r1t,r2t,r3t,r4t)
M = [0 -3.8462 0;4.4412 2.2206 0;-1.5702 -3.3140 -4.7104];
R = [r2t^2-r1t^2;r3t^2-r2t^2;r4t^2-r3t^2];
P = M*R;
x = P(1);
y = P(2);
z = P(3);

== matlab function Unknown_Terrain_BOTS/BOT4/Pose Estimator Bot4 ==
  data: x output; r1t input; y output; r2t input; r3t input; r4t input; z output
function [x,y,z] = fcn(r1t,r2t,r3t,r4t)
M = [0 -3.8462 0;4.4412 2.2206 0;-1.5702 -3.3140 -4.7104];
R = [r2t^2-r1t^2;r3t^2-r2t^2;r4t^2-r3t^2];
P = M*R;
x = P(1);
y = P(2);
z = P(3);

== matlab function Unknown_Terrain_BOTS/BOT4/Receiver1 ==
  data: x1 input; ed1 output; y1 input; z1 input; x2 input; y2 input; z2 input; x3 input; y3 input; z3 input; x4 input; y4 input; z4 input; ed2 output; ed3 output; ed4 output
function [ed1,ed2,ed3,ed4] = fcn(x1,y1,z1,x2,y2,z2,x3,y3,z3,x4,y4,z4)
ed1 = ((x1-x4)^2+(y1-0.57735-y4)^2+(z1+0.204124-z4)^2)^0.5;
ed2 = ((x2-x4)^2+(y2-0.57735-y4)^2+(z2+0.204124-z4)^2)^0.5;
ed3 = ((x3-x4)^2+(y3-0.57735-y4)^2+(z3+0.204124-z4)^2)^0.5;
ed4 = ((x4-x4)^2+(y4-0.57735-y4)^2+(z4+0.204124-z4)^2)^0.5;

== matlab function Unknown_Terrain_BOTS/BOT4/Receiver2 ==
  data: x1 input; ed1 output; y1 input; z1 input; x2 input; y2 input; z2 input; x3 input; y3 input; z3 input; x4 input; y4 input; z4 input; ed2 output; ed3 output; ed4 output
function [ed1,ed2,ed3,ed4] = fcn(x1,y1,z1,x2,y2,z2,x3,y3,z3,x4,y4,z4)
ed1 = ((x1+0.5-x4)^2+(y1+0.28867-y4)^2+(z1+0.204124-z4)^2)^0.5;
ed2 = ((x2+0.5-x4)^2+(y2+0.28867-y4)^2+(z2+0.204124-z4)^2)^0.5;
ed3 = ((x3+0.5-x4)^2+(y3+0.28867-y4)^2+(z3+0.204124-z4)^2)^0.5;
ed4 = ((x4+0.5-x4)^2+(y4+0.28867-y4)^2+(z4+0.204124-z4)^2)^0.5;

== matlab function Unknown_Terrain_BOTS/BOT4/Receiver3 ==
  data: x1 input; ed1 output; y1 input; z1 input; x2 input; y2 input; z2 input; x3 input; y3 input; z3 input; x4 input; y4 input; z4 input; ed2 output; ed3 output; ed4 output
function [ed1,ed2,ed3,ed4] = fcn(x1,y1,z1,x2,y2,z2,x3,y3,z3,x4,y4,z4)
ed1 = ((x1-0.5-x4)^2+(y1+0.28867-y4)^2+(z1+0.204124-z4)^2)^0.5;
ed2 = ((x2-0.5-x4)^2+(y2+0.28867-y4)^2+(z2+0.204124-z4)^2)^0.5;
ed3 = ((x3-0.5-x4)^2+(y3+0.28867-y4)^2+(z3+0.204124-z4)^2)^0.5;
ed4 = ((x4-0.5-x4)^2+(y4+0.28867-y4)^2+(z4+0.204124-z4)^2)^0.5;

== matlab function Unknown_Terrain_BOTS/BOT4/Receiver4 ==
  data: x1 input; ed1 output; y1 input; z1 input; x2 input; y2 input; z2 input; x3 input; y3 input; z3 input; x4 input; y4 input; z4 input; ed2 output; ed3 output; ed4 output
function [ed1,ed2,ed3,ed4] = fcn(x1,y1,z1,x2,y2,z2,x3,y3,z3,x4,y4,z4)
ed1 = ((x1-x4)^2+(y1-y4)^2+(z1+0.612372-z4)^2)^0.5;
ed2 = ((x2-x4)^2+(y2-y4)^2+(z2+0.612372-z4)^2)^0.5;
ed3 = ((x3-x4)^2+(y3-y4)^2+(z3+0.612372-z4)^2)^0.5;
ed4 = ((x4-x4)^2+(y4-y4)^2+(z4+0.612372-z4)^2)^0.5;

== matlab function Unknown_Terrain_BOTS/BOT1/Pose Estimator Bot1 ==
  data: x output; r1t input; y output; r2t input; r3t input; r4t input; z output
function [x,y,z] = fcn(r1t,r2t,r3t,r4t)
M = [0 -3.8462 0;4.4412 2.2206 0;-1.5702 -3.3140 -4.7104];
R = [r2t^2-r1t^2;r3t^2-r2t^2;r4t^2-r3t^2];
P = M*R;
x = P(1);
y = P(2);
z = P(3);

== matlab function Unknown_Terrain_BOTS/BOT1/Pose Estimator Bot2 ==
  data: x output; r1t input; y output; r2t input; r3t input; r4t input; z output
function [x,y,z] = fcn(r1t,r2t,r3t,r4t)
M = [0 -3.8462 0;4.4412 2.2206 0;-1.5702 -3.3140 -4.7104];
R = [r2t^2-r1t^2;r3t^2-r2t^2;r4t^2-r3t^2];
P = M*R;
x = P(1);
y = P(2);
z = P(3);

== matlab function Unknown_Terrain_BOTS/BOT1/Pose Estimator Bot3 ==
  data: x output; r1t input; y output; r2t input; r3t input; r4t input; z output
function [x,y,z] = fcn(r1t,r2t,r3t,r4t)
M = [0 -3.8462 0;4.4412 2.2206 0;-1.5702 -3.3140 -4.7104];
R = [r2t^2-r1t^2;r3t^2-r2t^2;r4t^2-r3t^2];
P = M*R;
x = P(1);
y = P(2);
z = P(3);

== matlab function Unknown_Terrain_BOTS/BOT1/Pose Estimator Bot4 ==
  data: x output; r1t input; y output; r2t input; r3t input; r4t input; z output
function [x,y,z] = fcn(r1t,r2t,r3t,r4t)
M = [0 -3.8462 0;4.4412 2.2206 0;-1.5702 -3.3140 -4.7104];
R = [r2t^2-r1t^2;r3t^2-r2t^2;r4t^2-r3t^2];
P = M*R;
x = P(1);
y = P(2);
z = P(3);

== matlab function Unknown_Terrain_BOTS/BOT1/Receiver1 ==
  data: x1 input; ed1 output; y1 input; z1 input; x2 input; y2 input; z2 input; x3 input; y3 input; z3 input; x4 input; y4 input; z4 input; ed2 output; ed3 output; ed4 output
function [ed1,ed2,ed3,ed4] = fcn(x1,y1,z1,x2,y2,z2,x3,y3,z3,x4,y4,z4)
ed1 = ((x1-x1)^2+(y1-0.57735-y1)^2+(z1+0.204124-z1)^2)^0.5;
ed2 = ((x2-x1)^2+(y2-0.57735-y1)^2+(z2+0.204124-z1)^2)^0.5;
ed3 = ((x3-x1)^2+(y3-0.57735-y1)^2+(z3+0.204124-z1)^2)^0.5;
ed4 = ((x4-x1)^2+(y4-0.57735-y1)^2+(z4+0.204124-z1)^2)^0.5;

== matlab function Unknown_Terrain_BOTS/BOT1/Receiver2 ==
  data: x1 input; ed1 output; y1 input; z1 input; x2 input; y2 input; z2 input; x3 input; y3 input; z3 input; x4 input; y4 input; z4 input; ed2 output; ed3 output; ed4 output
function [ed1,ed2,ed3,ed4] = fcn(x1,y1,z1,x2,y2,z2,x3,y3,z3,x4,y4,z4)
ed1 = ((x1+0.5-x1)^2+(y1+0.28867-y1)^2+(z1+0.204124-z1)^2)^0.5;
ed2 = ((x2+0.5-x1)^2+(y2+0.28867-y1)^2+(z2+0.204124-z1)^2)^0.5;
ed3 = ((x3+0.5-x1)^2+(y3+0.28867-y1)^2+(z3+0.204124-z1)^2)^0.5;
ed4 = ((x4+0.5-x1)^2+(y4+0.28867-y1)^2+(z4+0.204124-z1)^2)^0.5;

== matlab function Unknown_Terrain_BOTS/BOT1/Receiver3 ==
  data: x1 input; ed1 output; y1 input; z1 input; x2 input; y2 input; z2 input; x3 input; y3 input; z3 input; x4 input; y4 input; z4 input; ed2 output; ed3 output; ed4 output
function [ed1,ed2,ed3,ed4] = fcn(x1,y1,z1,x2,y2,z2,x3,y3,z3,x4,y4,z4)
ed1 = ((x1-0.5-x1)^2+(y1+0.28867-y1)^2+(z1+0.204124-z1)^2)^0.5;
ed2 = ((x2-0.5-x1)^2+(y2+0.28867-y1)^2+(z2+0.204124-z1)^2)^0.5;
ed3 = ((x3-0.5-x1)^2+(y3+0.28867-y1)^2+(z3+0.204124-z1)^2)^0.5;
ed4 = ((x4-0.5-x1)^2+(y4+0.28867-y1)^2+(z4+0.204124-z1)^2)^0.5;

== matlab function Unknown_Terrain_BOTS/BOT1/Receiver4 ==
  data: x1 input; ed1 output; y1 input; z1 input; x2 input; y2 input; z2 input; x3 input; y3 input; z3 input; x4 input; y4 input; z4 input; ed2 output; ed3 output; ed4 output
function [ed1,ed2,ed3,ed4] = fcn(x1,y1,z1,x2,y2,z2,x3,y3,z3,x4,y4,z4)
ed1 = ((x1-x1)^2+(y1-y1)^2+(z1+0.612372-z1)^2)^0.5;
ed2 = ((x2-x1)^2+(y2-y1)^2+(z2+0.612372-z1)^2)^0.5;
ed3 = ((x3-x1)^2+(y3-y1)^2+(z3+0.612372-z1)^2)^0.5;
ed4 = ((x4-x1)^2+(y4-y1)^2+(z4+0.612372-z1)^2)^0.5;

== matlab function Unknown_Terrain_BOTS/BOT2/Pose Estimator Bot1 ==
  data: x output; r1t input; y output; r2t input; r3t input; r4t input; z output
function [x,y,z] = fcn(r1t,r2t,r3t,r4t)
M = [0 -3.8462 0;4.4412 2.2206 0;-1.5702 -3.3140 -4.7104];
R = [r2t^2-r1t^2;r3t^2-r2t^2;r4t^2-r3t^2];
P = M*R;
x = P(1);
y = P(2);
z = P(3);

== matlab function Unknown_Terrain_BOTS/BOT2/Pose Estimator Bot2 ==
  data: x output; r1t input; y output; r2t input; r3t input; r4t input; z output
function [x,y,z] = fcn(r1t,r2t,r3t,r4t)
M = [0 -3.8462 0;4.4412 2.2206 0;-1.5702 -3.3140 -4.7104];
R = [r2t^2-r1t^2;r3t^2-r2t^2;r4t^2-r3t^2];
P = M*R;
x = P(1);
y = P(2);
z = P(3);

== matlab function Unknown_Terrain_BOTS/BOT2/Pose Estimator Bot3 ==
  data: x output; r1t input; y output; r2t input; r3t input; r4t input; z output
function [x,y,z] = fcn(r1t,r2t,r3t,r4t)
M = [0 -3.8462 0;4.4412 2.2206 0;-1.5702 -3.3140 -4.7104];
R = [r2t^2-r1t^2;r3t^2-r2t^2;r4t^2-r3t^2];
P = M*R;
x = P(1);
y = P(2);
z = P(3);

== matlab function Unknown_Terrain_BOTS/BOT2/Pose Estimator Bot4 ==
  data: x output; r1t input; y output; r2t input; r3t input; r4t input; z output
function [x,y,z] = fcn(r1t,r2t,r3t,r4t)
M = [0 -3.8462 0;4.4412 2.2206 0;-1.5702 -3.3140 -4.7104];
R = [r2t^2-r1t^2;r3t^2-r2t^2;r4t^2-r3t^2];
P = M*R;
x = P(1);
y = P(2);
z = P(3);

== matlab function Unknown_Terrain_BOTS/BOT2/Receiver1 ==
  data: x1 input; ed1 output; y1 input; z1 input; x2 input; y2 input; z2 input; x3 input; y3 input; z3 input; x4 input; y4 input; z4 input; ed2 output; ed3 output; ed4 output
function [ed1,ed2,ed3,ed4] = fcn(x1,y1,z1,x2,y2,z2,x3,y3,z3,x4,y4,z4)
ed1 = ((x1-x2)^2+(y1-0.57735-y2)^2+(z1+0.204124-z2)^2)^0.5;
ed2 = ((x2-x2)^2+(y2-0.57735-y2)^2+(z2+0.204124-z2)^2)^0.5;
ed3 = ((x3-x2)^2+(y3-0.57735-y2)^2+(z3+0.204124-z2)^2)^0.5;
ed4 = ((x4-x2)^2+(y4-0.57735-y2)^2+(z4+0.204124-z2)^2)^0.5;

== matlab function Unknown_Terrain_BOTS/BOT2/Receiver2 ==
  data: x1 input; ed1 output; y1 input; z1 input; x2 input; y2 input; z2 input; x3 input; y3 input; z3 input; x4 input; y4 input; z4 input; ed2 output; ed3 output; ed4 output
function [ed1,ed2,ed3,ed4] = fcn(x1,y1,z1,x2,y2,z2,x3,y3,z3,x4,y4,z4)
ed1 = ((x1+0.5-x2)^2+(y1+0.28867-y2)^2+(z1+0.204124-z2)^2)^0.5;
ed2 = ((x2+0.5-x2)^2+(y2+0.28867-y2)^2+(z2+0.204124-z2)^2)^0.5;
ed3 = ((x3+0.5-x2)^2+(y3+0.28867-y2)^2+(z3+0.204124-z2)^2)^0.5;
ed4 = ((x4+0.5-x2)^2+(y4+0.28867-y2)^2+(z4+0.204124-z2)^2)^0.5;

== matlab function Unknown_Terrain_BOTS/BOT2/Receiver3 ==
  data: x1 input; ed1 output; y1 input; z1 input; x2 input; y2 input; z2 input; x3 input; y3 input; z3 input; x4 input; y4 input; z4 input; ed2 output; ed3 output; ed4 output
function [ed1,ed2,ed3,ed4] = fcn(x1,y1,z1,x2,y2,z2,x3,y3,z3,x4,y4,z4)
ed1 = ((x1-0.5-x2)^2+(y1+0.28867-y2)^2+(z1+0.204124-z2)^2)^0.5;
ed2 = ((x2-0.5-x2)^2+(y2+0.28867-y2)^2+(z2+0.204124-z2)^2)^0.5;
ed3 = ((x3-0.5-x2)^2+(y3+0.28867-y2)^2+(z3+0.204124-z2)^2)^0.5;
ed4 = ((x4-0.5-x2)^2+(y4+0.28867-y2)^2+(z4+0.204124-z2)^2)^0.5;

== matlab function Unknown_Terrain_BOTS/BOT2/Receiver4 ==
  data: x1 input; ed1 output; y1 input; z1 input; x2 input; y2 input; z2 input; x3 input; y3 input; z3 input; x4 input; y4 input; z4 input; ed2 output; ed3 output; ed4 output
function [ed1,ed2,ed3,ed4] = fcn(x1,y1,z1,x2,y2,z2,x3,y3,z3,x4,y4,z4)
ed1 = ((x1-x2)^2+(y1-y2)^2+(z1+0.612372-z2)^2)^0.5;
ed2 = ((x2-x2)^2+(y2-y2)^2+(z2+0.612372-z2)^2)^0.5;
ed3 = ((x3-x2)^2+(y3-y2)^2+(z3+0.612372-z2)^2)^0.5;
ed4 = ((x4-x2)^2+(y4-y2)^2+(z4+0.612372-z2)^2)^0.5;

== matlab function Unknown_Terrain_BOTS/BOT3/Pose Estimator Bot1 ==
  data: x output; r1t input; y output; r2t input; r3t input; r4t input; z output
function [x,y,z] = fcn(r1t,r2t,r3t,r4t)
M = [0 -3.8462 0;4.4412 2.2206 0;-1.5702 -3.3140 -4.7104];
R = [r2t^2-r1t^2;r3t^2-r2t^2;r4t^2-r3t^2];
P = M*R;
x = P(1);
y = P(2);
z = P(3);

== matlab function Unknown_Terrain_BOTS/BOT3/Pose Estimator Bot2 ==
  data: x output; r1t input; y output; r2t input; r3t input; r4t input; z output
function [x,y,z] = fcn(r1t,r2t,r3t,r4t)
M = [0 -3.8462 0;4.4412 2.2206 0;-1.5702 -3.3140 -4.7104];
R = [r2t^2-r1t^2;r3t^2-r2t^2;r4t^2-r3t^2];
P = M*R;
x = P(1);
y = P(2);
z = P(3);

== matlab function Unknown_Terrain_BOTS/BOT3/Pose Estimator Bot3 ==
  data: x output; r1t input; y output; r2t input; r3t input; r4t input; z output
function [x,y,z] = fcn(r1t,r2t,r3t,r4t)
M = [0 -3.8462 0;4.4412 2.2206 0;-1.5702 -3.3140 -4.7104];
R = [r2t^2-r1t^2;r3t^2-r2t^2;r4t^2-r3t^2];
P = M*R;
x = P(1);
y = P(2);
z = P(3);

== matlab function Unknown_Terrain_BOTS/BOT3/Pose Estimator Bot4 ==
  data: x output; r1t input; y output; r2t input; r3t input; r4t input; z output
function [x,y,z] = fcn(r1t,r2t,r3t,r4t)
M = [0 -3.8462 0;4.4412 2.2206 0;-1.5702 -3.3140 -4.7104];
R = [r2t^2-r1t^2;r3t^2-r2t^2;r4t^2-r3t^2];
P = M*R;
x = P(1);
y = P(2);
z = P(3);

== matlab function Unknown_Terrain_BOTS/BOT3/Receiver1 ==
  data: x1 input; ed1 output; y1 input; z1 input; x2 input; y2 input; z2 input; x3 input; y3 input; z3 input; x4 input; y4 input; z4 input; ed2 output; ed3 output; ed4 output
function [ed1,ed2,ed3,ed4] = fcn(x1,y1,z1,x2,y2,z2,x3,y3,z3,x4,y4,z4)
ed1 = ((x1-x3)^2+(y1-0.57735-y3)^2+(z1+0.204124-z3)^2)^0.5;
ed2 = ((x2-x3)^2+(y2-0.57735-y3)^2+(z2+0.204124-z3)^2)^0.5;
ed3 = ((x3-x3)^2+(y3-0.57735-y3)^2+(z3+0.204124-z3)^2)^0.5;
ed4 = ((x4-x3)^2+(y4-0.57735-y3)^2+(z4+0.204124-z3)^2)^0.5;

== matlab function Unknown_Terrain_BOTS/BOT3/Receiver2 ==
  data: x1 input; ed1 output; y1 input; z1 input; x2 input; y2 input; z2 input; x3 input; y3 input; z3 input; x4 input; y4 input; z4 input; ed2 output; ed3 output; ed4 output
function [ed1,ed2,ed3,ed4] = fcn(x1,y1,z1,x2,y2,z2,x3,y3,z3,x4,y4,z4)
ed1 = ((x1+0.5-x3)^2+(y1+0.28867-y3)^2+(z1+0.204124-z3)^2)^0.5;
ed2 = ((x2+0.5-x3)^2+(y2+0.28867-y3)^2+(z2+0.204124-z3)^2)^0.5;
ed3 = ((x3+0.5-x3)^2+(y3+0.28867-y3)^2+(z3+0.204124-z3)^2)^0.5;
ed4 = ((x4+0.5-x3)^2+(y4+0.28867-y3)^2+(z4+0.204124-z3)^2)^0.5;

== matlab function Unknown_Terrain_BOTS/BOT3/Receiver3 ==
  data: x1 input; ed1 output; y1 input; z1 input; x2 input; y2 input; z2 input; x3 input; y3 input; z3 input; x4 input; y4 input; z4 input; ed2 output; ed3 output; ed4 output
function [ed1,ed2,ed3,ed4] = fcn(x1,y1,z1,x2,y2,z2,x3,y3,z3,x4,y4,z4)
ed1 = ((x1-0.5-x3)^2+(y1+0.28867-y3)^2+(z1+0.204124-z3)^2)^0.5;
ed2 = ((x2-0.5-x3)^2+(y2+0.28867-y3)^2+(z2+0.204124-z3)^2)^0.5;
ed3 = ((x3-0.5-x3)^2+(y3+0.28867-y3)^2+(z3+0.204124-z3)^2)^0.5;
ed4 = ((x4-0.5-x3)^2+(y4+0.28867-y3)^2+(z4+0.204124-z3)^2)^0.5;

== matlab function Unknown_Terrain_BOTS/BOT3/Receiver4 ==
  data: x1 input; ed1 output; y1 input; z1 input; x2 input; y2 input; z2 input; x3 input; y3 input; z3 input; x4 input; y4 input; z4 input; ed2 output; ed3 output; ed4 output
function [ed1,ed2,ed3,ed4] = fcn(x1,y1,z1,x2,y2,z2,x3,y3,z3,x4,y4,z4)
ed1 = ((x1-x3)^2+(y1-y3)^2+(z1+0.612372-z3)^2)^0.5;
ed2 = ((x2-x3)^2+(y2-y3)^2+(z2+0.612372-z3)^2)^0.5;
ed3 = ((x3-x3)^2+(y3-y3)^2+(z3+0.612372-z3)^2)^0.5;
ed4 = ((x4-x3)^2+(y4-y3)^2+(z4+0.612372-z3)^2)^0.5;
